simulink model "pilotInterface"  (Simulink 8.4)
settings: Solver=ode45  StartTime=0.0  StopTime=10.0  RelTol=1e-3
settings Model: Creator=brtaylor  LastModifiedBy=brtaylor
settings DataIOCC: SignalLoggingSaveFormat=Dataset
settings OptimizationCC: ExpressionDepthLimit=128
settings DebuggingCC: UnderspecifiedInitializationDetection=Simplified  MergeDetectMultiDrivingBlocksExec=error  FcnCallInpInsideContextMsg=EnableAllAsError  StateNameClashWarn=none
settings GRTTargetCC: CombineOutputUpdateFcns=on  GRTInterface=off

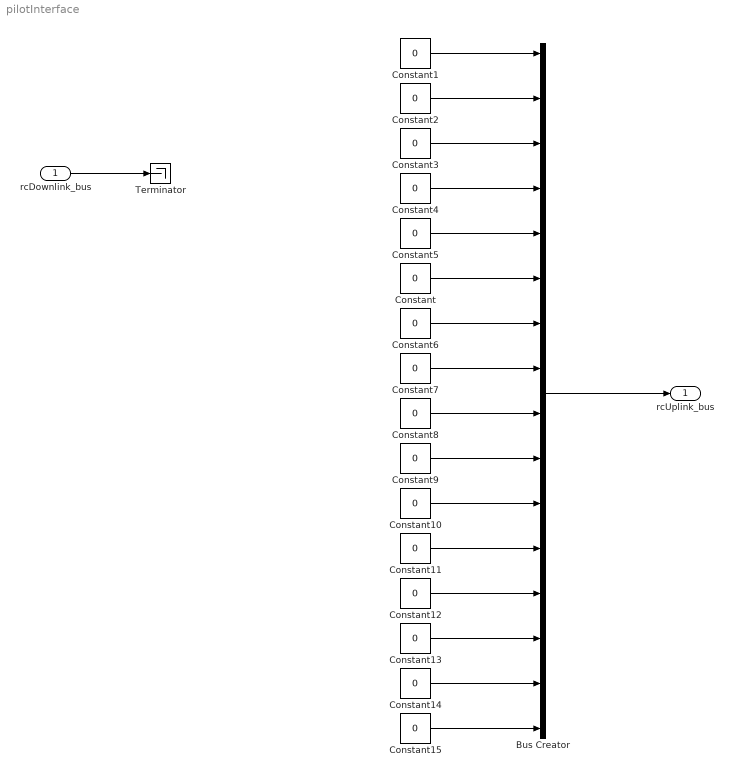
== system pilotInterface ==
  rcDownlink_bus : Inport
  Bus Creator : BusCreator  Inputs=16
  Constant{,1..15} (16 alike) : Constant  Value=0
  Terminator : Terminator
  rcUplink_bus : Outport
  wires:
  rcDownlink_bus/1 -> Terminator/1
  Bus Creator/1 -> rcUplink_bus/1
  Constant1/1 -> Bus Creator/1
  Constant5/1 -> Bus Creator/5
  Constant11/1 -> Bus Creator/12
  Constant6/1 -> Bus Creator/7
  Constant9/1 -> Bus Creator/10
  Constant2/1 -> Bus Creator/2
  Constant/1 -> Bus Creator/6
  Constant10/1 -> Bus Creator/11
  Constant13/1 -> Bus Creator/14
  Constant4/1 -> Bus Creator/4
  Constant12/1 -> Bus Creator/13
  Constant14/1 -> Bus Creator/15
  Constant15/1 -> Bus Creator/16
  Constant7/1 -> Bus Creator/8
  Constant8/1 -> Bus Creator/9
  Constant3/1 -> Bus Creator/3
